simulink model "Der_Faux_FPGA_V2_optimized_synthesizable"  (R2020a)
settings: Solver=FixedStepDiscrete  StartTime=0.0  StopTime=0.84375  FixedStep=1/fs_sim  RelTol=1e-3
values from neighbouring files (symbols this model uses):
  ADC_res = 5    [Der_Faux_ctr_FPGA.m]
  ADC_res_G4 = 8    [Der_Faux_ctr_FPGA.m]
  fs = 48000    [Der_Faux_ctr_FPGA.m]
  fs_sim = fs*ovs    (= 6144000)    [Der_Faux_ctr_FPGA.m]
  Gvar1_N = fi(Gvar1_N,0,ADC_res,0)    [Der_Faux_ctr_FPGA.m]
  Gvar2_N = fi(Gvar2_N,0,ADC_res,0)    [Der_Faux_ctr_FPGA.m]
  Gvar3_N = fi(Gvar3_N,0,ADC_res,0)    [Der_Faux_ctr_FPGA.m]
  Gvar4_N = fi(Gvar4_N,0,ADC_res_G4,0)    [Der_Faux_ctr_FPGA.m]
  input_space = linspace(0,2^ADC_res-1,2^ADC_res)    [Der_Faux_ctr_FPGA.m]
  input_spcae_extended = linspace(0,(2^ADC_res)^3-1,(2^ADC_res)^3)    [Der_Faux_ctr_FPGA.m]
  LUT_Z22a_opt = sfi(LUT_Z22a, len_LUT22a)    [Der_Faux_ctr_FPGA.m]
  LUT_Z22b_opt = sfi(LUT_Z22b, len_LUT22b)    [Der_Faux_ctr_FPGA.m]
  LUT_Z23a_opt = sfi(LUT_Z23a, len_Z23a)    [Der_Faux_ctr_FPGA.m]
  LUT_Z23b_opt = sfi(LUT_Z23b, len_Z23b)    [Der_Faux_ctr_FPGA.m]
  LUT_Z24a_opt = sfi(LUT_Z24a, len_LUT24a)    [Der_Faux_ctr_FPGA.m]
  LUT_Z24b_opt = sfi(LUT_Z24b, len_LUT24b)    [Der_Faux_ctr_FPGA.m]
  LUT_Z25a_opt = sfi(LUT_Z25a, len_LUT25a)    [Der_Faux_ctr_FPGA.m]
  LUT_Z25b_opt = sfi(LUT_Z25b, len_LUT25b)    [Der_Faux_ctr_FPGA.m]
  shift_reg_size = 8*44000    (= 352000)    [Der_Faux_ctr_FPGA.m]
  use_stimuli = [true,true,true,true]    [Der_Faux_ctr_FPGA.m]
  WL_RAM = 5    [Der_Faux_ctr_FPGA.m]
undefined symbols (not defined in the file or in its folder): poti_stimuli1, poti_stimuli2, poti_stimuli3, poti_stimuli4
libraries: hdlmdlgenlib x30, simulink x6, hdlsllib x4
(part 1 of 3)
settings Model: Creator=Donut  LastModifiedBy=Donut
settings OptimizationCC: BlockReduction=off  ConditionallyExecuteInputs=off  DefaultParameterBehavior=Inlined
settings DebuggingCC: SignalRangeChecking=warning  AlgebraicLoopMsg=error  InheritedTsInSrcMsg=none  SingleTaskRateTransMsg=error  ParameterOverflowMsg=warning  ParameterUnderflowMsg=warning  UnnecessaryDatatypeConvMsg=warning
settings HardwareCC: ProdBitPerPointer=32  ProdBitPerSizeT=32  ProdBitPerPtrDiffT=32  ProdLargestAtomicFloat=None  ProdIntDivRoundTo=Undefined  ProdEndianess=Unspecified  ProdWordSize=32  ProdHWDeviceType=ASIC/FPGA->ASIC/FPGA  TargetBitPerPointer=64  TargetBitPerSizeT=64  TargetBitPerPtrDiffT=64  TargetLongLongMode=on  TargetIntDivRoundTo=Zero  TargetEndianess=LittleEndian  TargetWordSize=64  TargetHWDeviceType=Custom Processor->MATLAB Host Computer  ProdEqTarget=off
settings SFSimCC: CustomCodeUndefinedFunction=UseInterfaceOnly

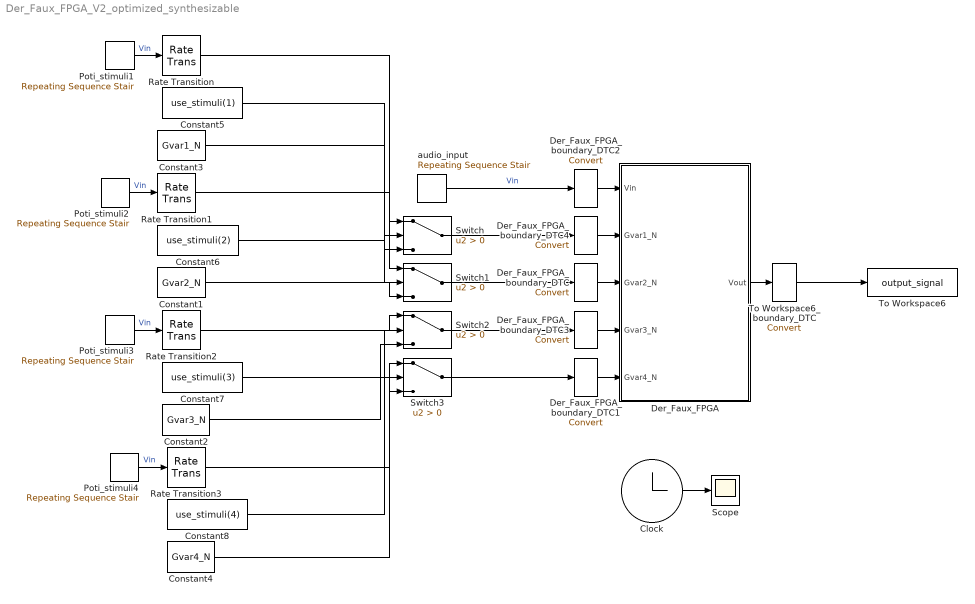
== system Der_Faux_FPGA_V2_optimized_synthesizable ==
  Clock : Clock
  Constant1 : Constant  Value=Gvar2_N  OutDataTypeStr=fixdt(0,ADC_res,0)  SampleTime=1/fs_sim  LockScale=on
  Constant2 : Constant  Value=Gvar3_N  OutDataTypeStr=fixdt(0,ADC_res,0)  SampleTime=1/fs_sim  LockScale=on
  Constant3 : Constant  Value=Gvar1_N  OutDataTypeStr=fixdt(0,ADC_res,0)  SampleTime=1/fs_sim  LockScale=on
  Constant4 : Constant  Value=Gvar4_N  OutDataTypeStr=fixdt(0,ADC_res_G4,0)  SampleTime=1/(fs_sim)  LockScale=on
  Constant5 : Constant  Value=use_stimuli(1)  OutDataTypeStr=boolean  SampleTime=1/fs_sim  LockScale=on
  Constant6 : Constant  Value=use_stimuli(2)  OutDataTypeStr=boolean  SampleTime=1/fs_sim  LockScale=on
  Constant7 : Constant  Value=use_stimuli(3)  OutDataTypeStr=boolean  SampleTime=1/fs_sim  LockScale=on
  Constant8 : Constant  Value=use_stimuli(4)  OutDataTypeStr=boolean  SampleTime=1/(fs_sim)  LockScale=on
  Der_Faux_FPGA : Subsystem
  Der_Faux_FPGA_boundary_DTC{,1..4} (5 alike) : DataTypeConversion  SaturateOnIntegerOverflow=on  RndMeth=Zero
  "Poti_stimuli1 " : simulink/Sources/Repeating Sequence Stair  OutValues=poti_stimuli1'  tsamp=1/fs  OutMin=[]  OutMax=[]  OutDataTypeStr=fixdt(0,ADC_res,0)  OutputDataTypeScalingMode=Specify via dialog  OutDataType=fixdt(0,ADC_res,0)  ConRadixGroup=Best Precision: Vector-wise  OutScaling=[]
      settings: LockScale=on
  "Poti_stimuli2 " : simulink/Sources/Repeating Sequence Stair  OutValues=poti_stimuli2'  tsamp=1/fs  OutMin=[]  OutMax=[]  OutDataTypeStr=fixdt(0,ADC_res,0)  OutputDataTypeScalingMode=Specify via dialog  OutDataType=fixdt(0,ADC_res,0)  ConRadixGroup=Best Precision: Vector-wise  OutScaling=[]
      settings: LockScale=on
  Poti_stimuli3 : simulink/Sources/Repeating Sequence Stair  OutValues=poti_stimuli3'  tsamp=1/fs  OutMin=[]  OutMax=[]  OutDataTypeStr=fixdt(0,ADC_res,0)  OutputDataTypeScalingMode=Specify via dialog  OutDataType=fixdt(0,ADC_res,0)  ConRadixGroup=Best Precision: Vector-wise  OutScaling=[]
      settings: LockScale=on
  Poti_stimuli4 : simulink/Sources/Repeating Sequence Stair  OutValues=poti_stimuli4'  tsamp=1/fs  OutMin=[]  OutMax=[]  OutDataTypeStr=fixdt(0,ADC_res_G4,0)  OutputDataTypeScalingMode=Specify via dialog  OutDataType=fixdt(0,ADC_res_G4,0)  ConRadixGroup=Best Precision: Vector-wise  OutScaling=[]
      settings: LockScale=on
  Rate Transition{,1..3} (4 alike) : RateTransition  OutPortSampleTime=1/fs_sim
  Scope : Scope
  Switch : Switch  Criteria=u2 > Threshold  OutDataTypeStr=fixdt(0,ADC_res,0)
      settings: LockScale=on
  Switch1 : Switch  Criteria=u2 > Threshold  OutDataTypeStr=fixdt(0,ADC_res,0)
      settings: LockScale=on
  Switch2 : Switch  Criteria=u2 > Threshold  OutDataTypeStr=fixdt(0,ADC_res,0)
      settings: LockScale=on
  Switch3 : Switch  Criteria=u2 > Threshold  OutDataTypeStr=fixdt(0,ADC_res_G4,0)
      settings: LockScale=on
  To Workspace6 : ToWorkspace  VariableName=output_signal  SaveFormat=Timeseries  SampleTime=1/fs
  To Workspace6_boundary_DTC : DataTypeConversion  SaturateOnIntegerOverflow=on  RndMeth=Zero
  audio_input : simulink/Sources/Repeating Sequence Stair  OutValues=audio'  tsamp=1/fs  OutMin=[]  OutMax=[]  OutDataTypeStr=fixdt(1,16,15)  OutputDataTypeScalingMode=Specify via dialog  OutDataType=fixdt(1,16,15)  ConRadixGroup=Best Precision: Vector-wise  OutScaling=[]
      settings: LockScale=on
  wires:
  Der_Faux_FPGA_boundary_DTC4/1 -> Der_Faux_FPGA/2(Gvar1_N)
  Switch/1 -> Der_Faux_FPGA_boundary_DTC4/1
  Der_Faux_FPGA_boundary_DTC3/1 -> Der_Faux_FPGA/4(Gvar3_N)
  Switch2/1 -> Der_Faux_FPGA_boundary_DTC3/1
  Der_Faux_FPGA_boundary_DTC2/1 -> Der_Faux_FPGA/1(Vin)
  audio_input/1 -> Der_Faux_FPGA_boundary_DTC2/1  "Vin"
  Der_Faux_FPGA_boundary_DTC1/1 -> Der_Faux_FPGA/5(Gvar4_N)
  Switch3/1 -> Der_Faux_FPGA_boundary_DTC1/1
  Der_Faux_FPGA_boundary_DTC/1 -> Der_Faux_FPGA/3(Gvar2_N)
  Switch1/1 -> Der_Faux_FPGA_boundary_DTC/1
  To Workspace6_boundary_DTC/1 -> To Workspace6/1
  Der_Faux_FPGA/1(Vout) -> To Workspace6_boundary_DTC/1
  Rate Transition2/1 -> Switch2/1
  Rate Transition1/1 -> Switch1/1
  Poti_stimuli4/1 -> Rate Transition3/1  "Vin"
  Poti_stimuli3/1 -> Rate Transition2/1  "Vin"
  "Poti_stimuli2 "/1 -> Rate Transition1/1  "Vin"
  Rate Transition3/1 -> Switch3/1
  Rate Transition/1 -> Switch/1
  "Poti_stimuli1 "/1 -> Rate Transition/1  "Vin"
  Constant4/1 -> Switch3/3
  Constant2/1 -> Switch2/3
  Constant1/1 -> Switch1/3
  Constant3/1 -> Switch/3
  Constant7/1 -> Switch2/2
  Constant8/1 -> Switch3/2
  Constant6/1 -> Switch1/2
  Constant5/1 -> Switch/2
  Clock/1 -> Scope/1
